simulink model "adcs_sim_main_HIL"  (R2016b)
settings: Solver=VariableStepAuto  StartTime=0.0  StopTime=5400  RelTol=1e-3  EnableMultiTasking=on
InitFcn:
  | %sim_init
StopFcn:
  | %% SIM %%
  | 
  | % Extract States
  | states = logsout.getElement('states').Values;
  | quat = states.quaternion;
  | omega_radps = states.body_rates_radps;
  | pos_eci_km = states.position_eci_km;
  | vel_eci_kmps = states.velocity_eci_kmps;
  | 
  | % Extract Actuator measurements
  | act_meas = logsout.getElement('act_meas').Values;
  | 
  | % Extract Commands
  | cmds = logsout.getElement('commands').Values;
  | MT_dv = cmds.MT_dv;
  | 
  | % Extract sensor processing output
  | sp2fsw = logsout.getElement('sp2fsw').Values;
  | mag1_meas_T = sp2fsw.mag1_vec_body_T;
  | mag2_meas_T = sp2fsw.mag2_vec_body_T;
  | 
  | %% FSW %%
  | 
  | % CAN IN
  | canin = logsout.getElement('CAN_IN').Values;
  | sp2fsw = logsout.getElement('sp2fsw').Values;
  | 
  | % ENV ESTIM Output
  | env_estim = logsout.getElement('envest_2_fsw').Values;
  | sc_in_sun = env_estim.sc_in_sun;
  | sc_above_gs = env_estim.sc_above_gs;
  | sc_pos_eci_m = env_estim.pos_eci_m;
  | sc_vel_eci_mps = env_estim.vel_eci_mps;
  | 
  | % CAN OUT
  | canout = logsout.getElement('CAN_OUT').Values;
  | sc_quat = canout.sc_quat;
  | sc_omega_radps = canout.body_rates;
  | sc_mode = canout.sc_mode;
  | 
  | % Extract B-dot tumble status
  | cmd_bdot = logsout.getElement('cmd_MT_bdot').Values;
  | tumble = logsout.getElement('tumble').Values;
libraries: dynamics_lib x1, environment_lib x1, sensors_lib x1
settings Model: SimulationMode=accelerator  Creator=bbarz_000  LastModifiedBy=Taylor
settings DataIOCC: SaveOutput=off  DSMLogging=off
settings OptimizationCC: DefaultParameterBehavior=Inlined  UseDivisionForNetSlopeComputation=on  UseFloatMulNetSlope=on  InlineInvariantSignals=on  PassReuseOutputArgsAs=Individual arguments  ZeroExternalMemoryAtStartup=off  ZeroInternalMemoryAtStartup=off  NoFixptDivByZeroProtection=on  EfficientFloat2IntCast=on  LifeSpan=1
settings DebuggingCC: ReadBeforeWriteMsg=DisableAll  WriteAfterWriteMsg=DisableAll  WriteAfterReadMsg=DisableAll  MultiTaskDSMMsg=none  ParameterTunabilityLossMsg=error  SFUnexpectedBacktrackingDiag=warning  SFNoUnconditionalDefaultTransitionDiag=warning  SFExecutionAtInitializationDiag=none
settings HardwareCC: ProdBitPerInt=16  ProdBitPerPointer=16  ProdBitPerSizeT=16  ProdBitPerPtrDiffT=16  ProdLargestAtomicFloat=None  ProdWordSize=16  ProdHWDeviceType=Texas Instruments->MSP430
settings ModelReferenceCC: UpdateModelReferenceTargets=IfOutOfDate
settings SFSimCC: SFSimEcho=off
settings RTWCC: SystemTargetFile=ert.tlc  GenCodeOnly=on  PackageGeneratedCodeAndArtifacts=on  TemplateMakefile=ert_default_tmf  Description=Embedded Coder  GenerateReport=on  Toolchain=Clang v3.1 | gmake (64-bit Mac)  IncludeHyperlinkInReport=on  LaunchReport=on  GenerateTraceInfo=on  GenerateTraceReport=on  GenerateTraceReportSl=on  GenerateTraceReportSf=on  GenerateTraceReportEml=on  GenerateCodeMetricsReport=on
settings CodeAppCC: ForceParamTrailComments=on  IgnoreCustomStorageClasses=off  OperatorAnnotations=on  SimulinkDataObjDesc=on  SFDataObjDesc=on  MATLABFcnDesc=on  CustomSymbolStrGlobalVar=rt$N$M  CustomSymbolStrType=$N$M  CustomSymbolStrFcn=$N$M$F  CustomSymbolStrMacro=$N$M  InsertBlockDesc=on  MATLABSourceComments=on
settings ERTTargetCC: GenerateSampleERTMain=on  CombineSignalStateStructs=on  SupportComplex=off  SupportContinuousTime=on  SupportNonInlinedSFcns=on  InlinedParameterPlacement=NonHierarchical  ERTCustomFileTemplate=example_file_process.tlc  ERTFilePackagingFormat=CompactWithDataFile
settings ConfigComp: CovMetricSettings=dw  CovHtmlReporting=on  CovSaveCumulativeToWorkspaceVar=on  CovSaveSingleToWorkspaceVar=on  CovExternalEMLEnable=off

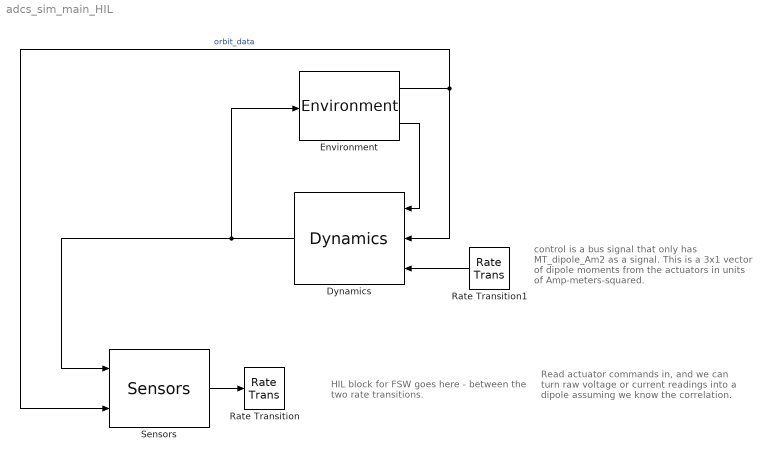
== system adcs_sim_main_HIL ==
  note: control is a bus signal that only has
      | MT_dipole_Am2 as a signal. This is a 3x1
      | vector of dipole moments from the actuators
      | in units of Amp-meters-squared.
  note: Read actuator commands in, and we can
      | turn raw voltage or current readings
      | into a dipole assuming we know the
      | correlation.
  note: HIL block for FSW goes here - between
      | the two rate transitions.
  Dynamics : dynamics_lib/Dynamics
  Environment : environment_lib/Environment
  Rate Transition : RateTransition  OutPortSampleTime=sim_params.HIL.sample_time_s
  Rate Transition1 : RateTransition
  Sensors : sensors_lib/Sensors
  wires:
  Dynamics/1 -> Environment/1, Sensors/1
  Environment/1 -> Sensors/2, Dynamics/2  "orbit_data"
  Rate Transition1/1 -> Dynamics/3
  Environment/2 -> Dynamics/1
  Sensors/1 -> Rate Transition/1
